simulink model "model_moment_bierny"  (Simulink 7.5)
settings: Solver=ode3  StartTime=0.0  StopTime=5  FixedStep=0.006  RelTol=1e-3
values from neighbouring files (symbols this model uses):
  J = Js + Jmr    [warunek.m]
  lambdaN = 2    [warunek.m]
  psien = (Un - Rt*In)/wn    [warunek.m]
  T = Lt/Rt    [warunek.m]
  wn = nn*2*pi/60    [warunek.m]
undefined symbols (not defined in the file or in its folder): In, Kp, Kt, Kw, m, Mn, Rt, Tr, Un, uz0, V, Y
settings Model: Creator=Konrad  LastModifiedBy=Konrad

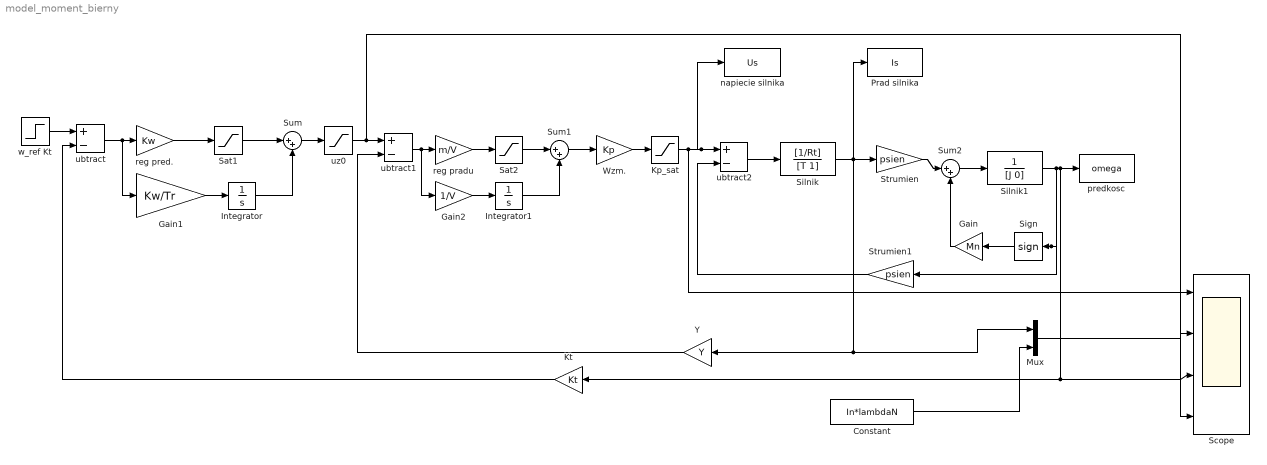
== system model_moment_bierny ==
  Constant : Constant  Value=In*lambdaN  OutDataType=fixdt(1, 16)  OutScaling=2^0
  Gain : Gain  Gain=Mn  ParameterDataType=fixdt(1, 16)  ParameterScaling=2^0  OutDataType=fixdt(1, 16)  OutScaling=2^0
  Gain1 : Gain  Gain=Kw/Tr  ParameterDataType=fixdt(1, 16)  ParameterScaling=2^0  OutDataType=fixdt(1, 16)  OutScaling=2^0
  Gain2 : Gain  Gain=1/V  ParameterDataType=fixdt(1, 16)  ParameterScaling=2^0  OutDataType=fixdt(1, 16)  OutScaling=2^0
  Integrator : Integrator  LimitOutput=on  UpperSaturationLimit=10  LowerSaturationLimit=-10
  Integrator1 : Integrator  LimitOutput=on  UpperSaturationLimit=10  LowerSaturationLimit=-10
  Kp_sat : Saturate  UpperLimit=1.5*Un  LowerLimit=-1.5*Un  OutDataType=fixdt(1, 16)  OutScaling=2^0
  Kt : Gain  Gain=Kt  ParameterDataType=fixdt(1, 16)  ParameterScaling=2^0  OutDataType=fixdt(1, 16)  OutScaling=2^0
  Mux : Mux  Inputs=2
  Prad silnika : ToWorkspace  VariableName=Is  SampleTime=-1  SaveFormat=Structure
  Sat1 : Saturate  UpperLimit=10  LowerLimit=-10  OutDataType=fixdt(1, 16)  OutScaling=2^0
  Sat2 : Saturate  UpperLimit=10  LowerLimit=-10  OutDataType=fixdt(1, 16)  OutScaling=2^0
  Scope : Scope  NumInputPorts=4
      settings: YMin=-5~-5~-5~-5  YMax=5~5~5~5
  Sign : Signum
  Silnik : TransferFcn  Numerator=[1/Rt]  Denominator=[T 1]
  Silnik1 : TransferFcn  Denominator=[J 0]
  Strumien : Gain  Gain=psien  ParameterDataType=fixdt(1, 16)  ParameterScaling=2^0  OutDataType=fixdt(1, 16)  OutScaling=2^0
  Strumien1 : Gain  Gain=psien  ParameterDataType=fixdt(1, 16)  ParameterScaling=2^0  OutDataType=fixdt(1, 16)  OutScaling=2^0
  Sum : Sum  Inputs=|++  OutDataType=fixdt(1, 16)  OutScaling=2^0
  Sum1 : Sum  Inputs=|++  OutDataType=fixdt(1, 16)  OutScaling=2^0
  Sum2 : Sum  Inputs=|++  OutDataType=fixdt(1, 16)  OutScaling=2^0
  Wzm. : Gain  Gain=Kp  ParameterDataType=fixdt(1, 16)  ParameterScaling=2^0  OutDataType=fixdt(1, 16)  OutScaling=2^0
  Y : Gain  Gain=Y  ParameterDataType=fixdt(1, 16)  ParameterScaling=2^0  OutDataType=fixdt(1, 16)  OutScaling=2^0
  napiecie silnika : ToWorkspace  VariableName=Us  SampleTime=-1  SaveFormat=Structure
  predkosc : ToWorkspace  VariableName=omega  SampleTime=-1  SaveFormat=Structure
  reg pradu : Gain  Gain=m/V  ParameterDataType=fixdt(1, 16)  ParameterScaling=2^0  OutDataType=fixdt(1, 16)  OutScaling=2^0
  reg pred. : Gain  Gain=Kw  ParameterDataType=fixdt(1, 16)  ParameterScaling=2^0  OutDataType=fixdt(1, 16)  OutScaling=2^0
  ubtract : Sum  Inputs=+-  OutDataType=fixdt(1, 16)  OutScaling=2^-10
  ubtract1 : Sum  Inputs=+-  OutDataType=fixdt(1, 16)  OutScaling=2^-10
  ubtract2 : Sum  Inputs=+-  OutDataType=fixdt(1, 16)  OutScaling=2^-10
  uz0 : Saturate  UpperLimit=uz0  LowerLimit=-uz0  OutDataType=fixdt(1, 16)  OutScaling=2^0
  w_ref Kt : Step  Time=0  After=wn*Kt  SampleTime=0
  wires:
  w_ref Kt/1 -> ubtract/1
  ubtract/1 -> reg pred./1, Gain1/1
  reg pred./1 -> Sat1/1
  Sat1/1 -> Sum/1
  Gain1/1 -> Integrator/1
  Integrator/1 -> Sum/2
  Sum/1 -> uz0/1
  uz0/1 -> ubtract1/1, Scope/4
  ubtract1/1 -> reg pradu/1, Gain2/1
  reg pradu/1 -> Sat2/1
  Sat2/1 -> Sum1/1
  Gain2/1 -> Integrator1/1
  Integrator1/1 -> Sum1/2
  Sum1/1 -> Wzm./1
  Wzm./1 -> Kp_sat/1
  Kp_sat/1 -> ubtract2/1, napiecie silnika/1, Scope/1
  ubtract2/1 -> Silnik/1
  Silnik/1 -> Strumien/1, Prad silnika/1, Mux/1, Y/1
  Strumien/1 -> Sum2/1
  Sum2/1 -> Silnik1/1
  Silnik1/1 -> predkosc/1, Scope/3, Kt/1, Strumien1/1, Sign/1
  Mux/1 -> Scope/2
  Strumien1/1 -> ubtract2/2
  Y/1 -> ubtract1/2
  Kt/1 -> ubtract/2
  Constant/1 -> Mux/2
  Gain/1 -> Sum2/2
  Sign/1 -> Gain/1
